simulink model "BlueROV2_Simu"  (R2023b)
settings: Solver=FixedStepAuto  StartTime=0.0  StopTime=60  FixedStep=dt  RelTol=1e-3
values from neighbouring files (symbols this model uses):
  dt = 0.1    [Integrate.m]    (also in init.m; init_NIF.m; init_NIF2.m; init_ODE.m)
  Opt_Ballast_Force = Ballast_Compute(Opt_Ballast_Config)    [init_ballast_checking.m]
  Param = BlueROV2_param()    [Integrate.m]    (also in init.m; init_NIF.m; init_NIF2.m; init_ODE.m)
  tau_b_test = [0; 0; 0; 0; 0; 0]    [init_ballast_checking.m]
  Tether_Force = zeros(6,1)    [Integrate.m]    (also in init.m; init_NIF.m; init_NIF2.m; init_ODE.m)
settings Model: Creator=goks  LastModifiedBy=HP

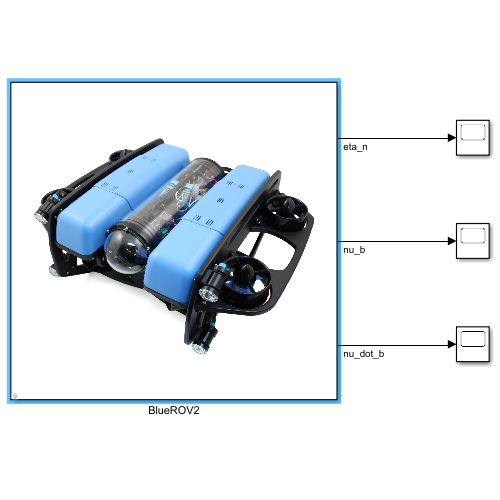
[thumbnail: Simulink's stored preview of the top-level diagram]
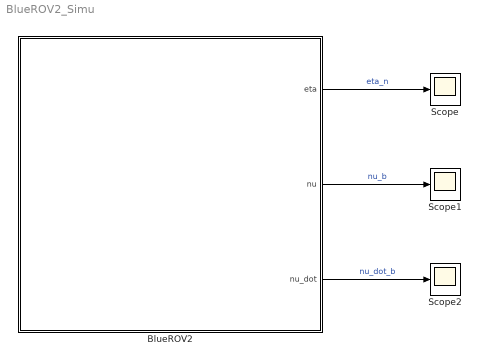
== system BlueROV2_Simu ==
  BlueROV2 : Subsystem
      mask DialogControl DescTextVar Prompt: %<BlueROV2>
      mask Display: image('heavy-bluerov.jpg');
  Scope : Scope
  Scope1 : Scope
  Scope2 : Scope
  wires:
  BlueROV2/1(eta) -> Scope/1  "eta_n"
  BlueROV2/2(nu) -> Scope1/1  "nu_b"
  BlueROV2/3(nu_dot) -> Scope2/1  "nu_dot_b"

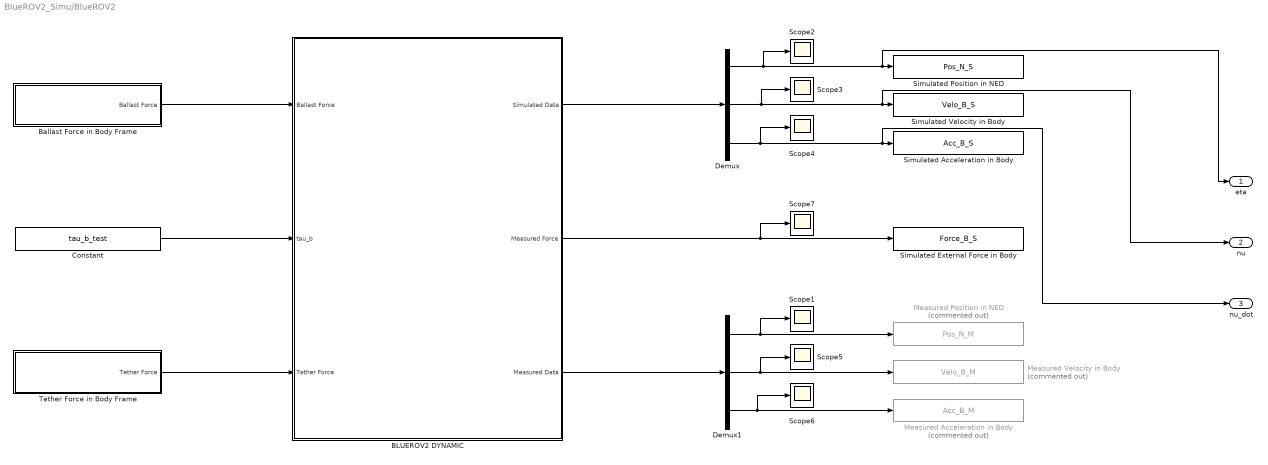
== system BlueROV2_Simu/BlueROV2 ==
  BLUEROV2 DYNAMIC : Subsystem
  Ballast Force in Body Frame : Subsystem
  Constant : Constant  Value=tau_b_test
  Demux : Demux  Outputs=3
  Demux1 : Demux  Outputs=3
  Measured Acceleration in Body : ToWorkspace  Commented=on  VariableName=Acc_B_M  SampleTime=-1
  Measured Position in NED : ToWorkspace  Commented=on  VariableName=Pos_N_M  SampleTime=-1
  Measured Velocity in Body : ToWorkspace  Commented=on  VariableName=Velo_B_M  SampleTime=-1
  Scope{1..7} (7 alike) : Scope
  Simulated Acceleration in Body : ToWorkspace  VariableName=Acc_B_S  SampleTime=-1
  Simulated External Force in Body : ToWorkspace  VariableName=Force_B_S  SampleTime=-1
  Simulated Position in NED : ToWorkspace  VariableName=Pos_N_S  SampleTime=-1
  Simulated Velocity in Body : ToWorkspace  VariableName=Velo_B_S  SampleTime=-1
  Tether Force in Body Frame : Subsystem
  eta : Outport
  nu : Outport  Port=2
  nu_dot : Outport  Port=3
  wires:
  Tether Force in Body Frame/1(Tether Force) -> BLUEROV2 DYNAMIC/3(Tether Force)
  Demux/2 -> Simulated Velocity in Body/1, nu/1, Scope3/1
  BLUEROV2 DYNAMIC/1(Simulated Data) -> Demux/1
  Demux1/1 -> Measured Position in NED/1, Scope1/1
  BLUEROV2 DYNAMIC/3(Measured Data) -> Demux1/1
  Ballast Force in Body Frame/1(Ballast Force) -> BLUEROV2 DYNAMIC/1(Ballast Force)
  Demux/1 -> eta/1, Simulated Position in NED/1, Scope2/1
  Demux1/2 -> Measured Velocity in Body/1, Scope5/1
  Demux1/3 -> Scope6/1, Measured Acceleration in Body/1
  BLUEROV2 DYNAMIC/2(Measured Force) -> Scope7/1, Simulated External Force in Body/1
  Constant/1 -> BLUEROV2 DYNAMIC/2(tau_b)
  Demux/3 -> nu_dot/1, Simulated Acceleration in Body/1, Scope4/1

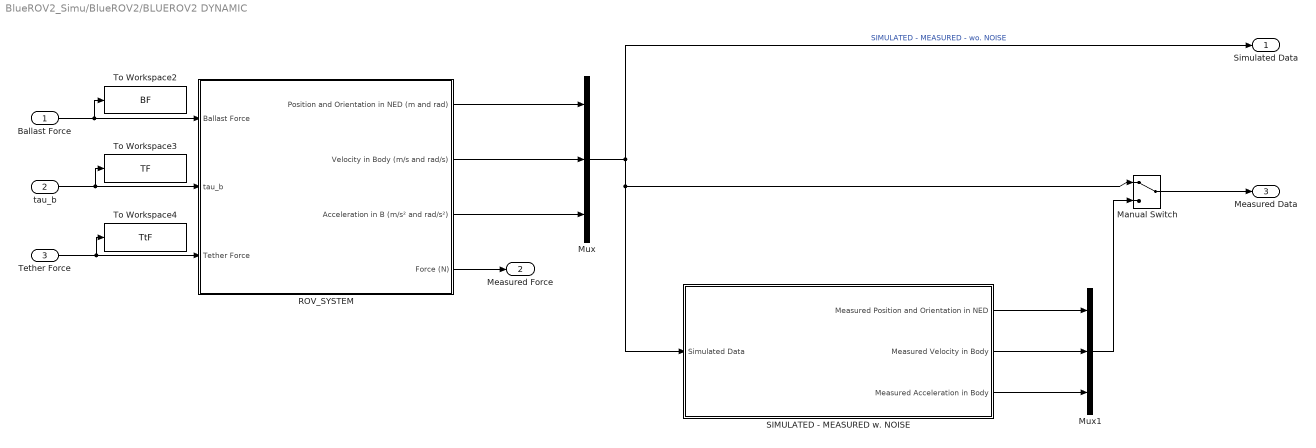
== system BlueROV2_Simu/BlueROV2/BLUEROV2 DYNAMIC ==
  Ballast Force : Inport
  tau_b : Inport  Port=2
  Tether Force : Inport  Port=3
  Manual Switch : ManualSwitch
  Mux : Mux  Inputs=3
  Mux1 : Mux  Inputs=3
  ROV_SYSTEM : Subsystem
  SIMULATED - MEASURED w. NOISE : Subsystem
  To Workspace2 : ToWorkspace  VariableName=BF  SampleTime=-1
  To Workspace3 : ToWorkspace  VariableName=TF  SampleTime=-1
  To Workspace4 : ToWorkspace  VariableName=TtF  SampleTime=-1
  Simulated Data : Outport
  Measured Force : Outport  Port=2
  Measured Data : Outport  Port=3
  wires:
  ROV_SYSTEM/1(Position and Orientation in NED (m and rad)) -> Mux/1
  ROV_SYSTEM/2(Velocity in Body (m/s and rad/s)) -> Mux/2
  ROV_SYSTEM/3(Acceleration in B (m/s² and rad/s²)) -> Mux/3
  ROV_SYSTEM/4(Force (N)) -> Measured Force/1
  SIMULATED - MEASURED w. NOISE/2(Measured Velocity in Body) -> Mux1/2
  SIMULATED - MEASURED w. NOISE/1(Measured Position and Orientation in NED) -> Mux1/1
  SIMULATED - MEASURED w. NOISE/3(Measured Acceleration in Body) -> Mux1/3
  Mux/1 -> SIMULATED - MEASURED w. NOISE/1(Simulated Data), Manual Switch/1, Simulated Data/1  "SIMULATED - MEASURED - wo. NOISE"
  Manual Switch/1 -> Measured Data/1
  Mux1/1 -> Manual Switch/2
  Ballast Force/1 -> ROV_SYSTEM/1(Ballast Force), To Workspace2/1
  tau_b/1 -> ROV_SYSTEM/2(tau_b), To Workspace3/1
  Tether Force/1 -> To Workspace4/1, ROV_SYSTEM/3(Tether Force)

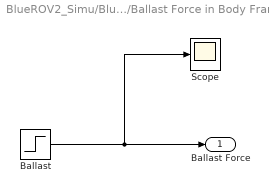
== system BlueROV2_Simu/BlueROV2/Ballast Force in Body Frame ==
  Ballast : Step  Time=0  Before=Opt_Ballast_Force  After=Opt_Ballast_Force  SampleTime=0
  Scope : Scope
  Ballast Force : Outport
  wires:
  Ballast/1 -> Scope/1, Ballast Force/1

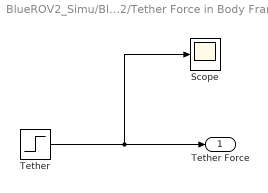
== system BlueROV2_Simu/BlueROV2/Tether Force in Body Frame ==
  Scope : Scope
  Tether : Step  Before=Tether_Force  After=Tether_Force  SampleTime=0
  Tether Force : Outport
  wires:
  Tether/1 -> Scope/1, Tether Force/1

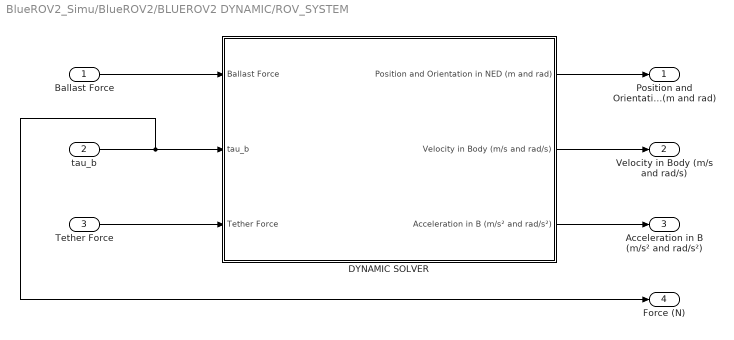
== system BlueROV2_Simu/BlueROV2/BLUEROV2 DYNAMIC/ROV_SYSTEM ==
  Ballast Force : Inport
  tau_b : Inport  Port=2
  Tether Force : Inport  Port=3
  DYNAMIC SOLVER : Subsystem
  Position and Orientation in NED (m and rad) : Outport
  Velocity in Body (m/s and rad/s) : Outport  Port=2
  Acceleration in B (m/s² and rad/s²) : Outport  Port=3
  Force (N) : Outport  Port=4
  wires:
  DYNAMIC SOLVER/2(Velocity in Body (m/s and rad/s)) -> Velocity in Body (m/s and rad/s)/1
  DYNAMIC SOLVER/1(Position and Orientation in NED (m and rad)) -> Position and Orientation in NED (m and rad)/1
  DYNAMIC SOLVER/3(Acceleration in B (m/s² and rad/s²)) -> Acceleration in B (m/s² and rad/s²)/1
  tau_b/1 -> DYNAMIC SOLVER/2(tau_b), Force (N)/1
  Ballast Force/1 -> DYNAMIC SOLVER/1(Ballast Force)
  Tether Force/1 -> DYNAMIC SOLVER/3(Tether Force)

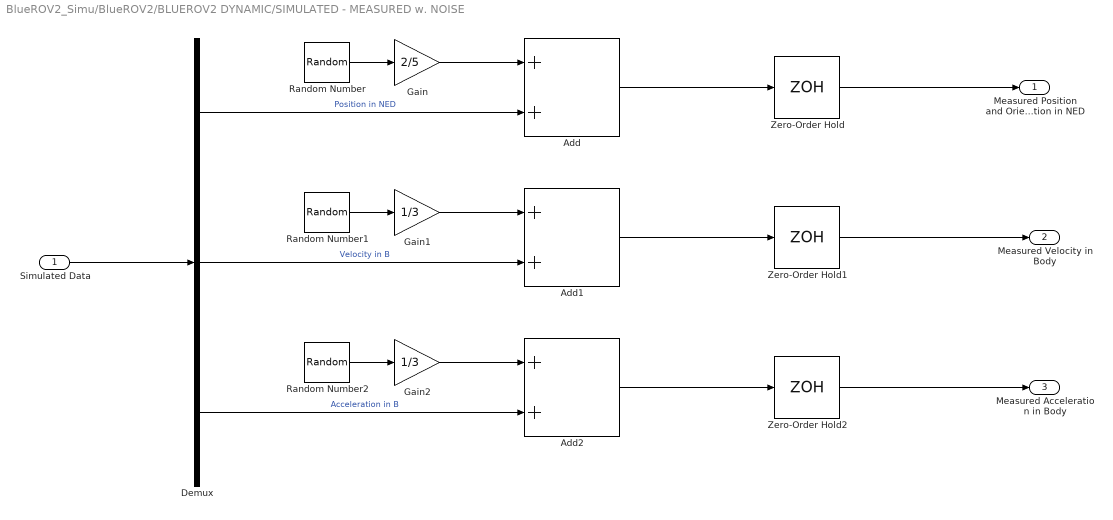
== system BlueROV2_Simu/BlueROV2/BLUEROV2 DYNAMIC/SIMULATED - MEASURED w. NOISE ==
  Simulated Data : Inport
  Add : Sum
  Add1 : Sum
  Add2 : Sum
  Demux : Demux  Outputs=3
  Gain : Gain  Gain=2/5
  Gain1 : Gain  Gain=1/3
  Gain2 : Gain  Gain=1/3
  Random Number : RandomNumber  Variance=0.01  SampleTime=dt
  Random Number1 : RandomNumber  Variance=0.01  SampleTime=dt
  Random Number2 : RandomNumber  Variance=0.01  SampleTime=dt
  Zero-Order Hold : ZeroOrderHold  SampleTime=-1
  Zero-Order Hold1 : ZeroOrderHold  SampleTime=-1
  Zero-Order Hold2 : ZeroOrderHold  SampleTime=-1
  Measured Position and Orientation in NED : Outport
  Measured Velocity in Body : Outport  Port=2
  Measured Acceleration in Body : Outport  Port=3
  wires:
  Simulated Data/1 -> Demux/1
  Demux/1 -> Add/2  "Position in NED"
  Random Number/1 -> Gain/1
  Gain/1 -> Add/1
  Random Number1/1 -> Gain1/1
  Demux/2 -> Add1/2  "Velocity in B"
  Gain1/1 -> Add1/1
  Random Number2/1 -> Gain2/1
  Demux/3 -> Add2/2  "Acceleration in B"
  Gain2/1 -> Add2/1
  Add/1 -> Zero-Order Hold/1
  Add1/1 -> Zero-Order Hold1/1
  Add2/1 -> Zero-Order Hold2/1
  Zero-Order Hold/1 -> Measured Position and Orientation in NED/1
  Zero-Order Hold1/1 -> Measured Velocity in Body/1
  Zero-Order Hold2/1 -> Measured Acceleration in Body/1

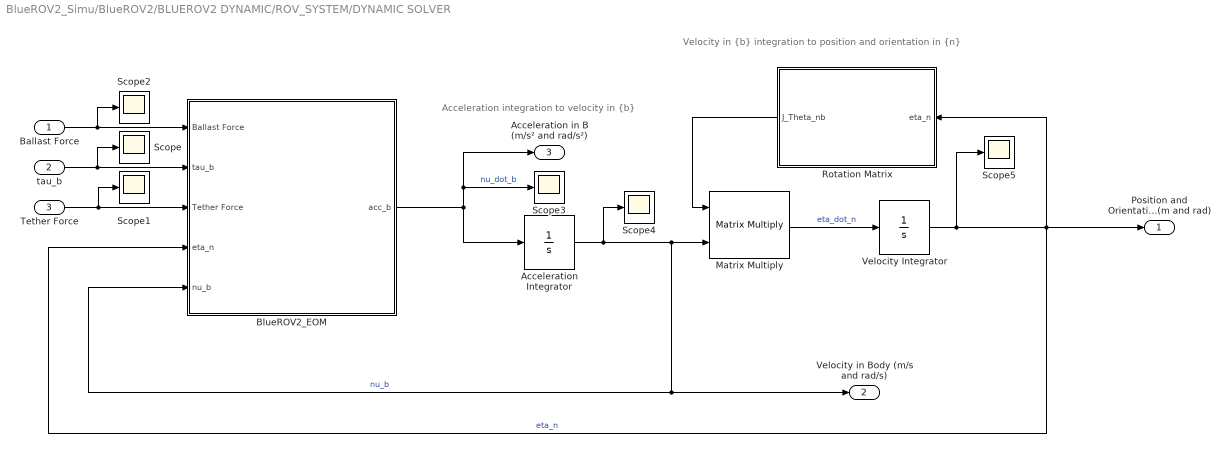
== system BlueROV2_Simu/BlueROV2/BLUEROV2 DYNAMIC/ROV_SYSTEM/DYNAMIC SOLVER ==
  note: Velocity in {b} integration to position and orientation in {n}
  note: Acceleration integration to velocity in {b}
  Ballast Force : Inport
  tau_b : Inport  Port=2
  Tether Force : Inport  Port=3
  Acceleration Integrator : Integrator  InitialCondition=Param.IC.Velo
  BlueROV2_EOM : Subsystem
  Matrix Multiply : Product  Multiplication=Matrix(*)
  Rotation Matrix : MATLAB Function  TreatAsAtomicUnit=on
  Scope{,1..5} (6 alike) : Scope
  Velocity Integrator : Integrator  InitialCondition=Param.IC.Pos
  Position and Orientation in NED (m and rad) : Outport
  Velocity in Body (m/s and rad/s) : Outport  Port=2
  Acceleration in B (m/s² and rad/s²) : Outport  Port=3
  wires:
  tau_b/1 -> BlueROV2_EOM/2(tau_b), Scope/1
  Rotation Matrix/1(J_Theta_nb) -> Matrix Multiply/1
  Matrix Multiply/1 -> Velocity Integrator/1  "eta_dot_n"
  Ballast Force/1 -> Scope2/1, BlueROV2_EOM/1(Ballast Force)
  BlueROV2_EOM/1(acc_b) -> Acceleration Integrator/1, Acceleration in B (m/s² and rad/s²)/1, Scope3/1  "nu_dot_b"
  Tether Force/1 -> BlueROV2_EOM/3(Tether Force), Scope1/1
  Velocity Integrator/1 -> BlueROV2_EOM/4(eta_n), Rotation Matrix/1(eta_n), Position and Orientation in NED (m and rad)/1, Scope5/1  "eta_n"
  Acceleration Integrator/1 -> Scope4/1, BlueROV2_EOM/5(nu_b), Velocity in Body (m/s and rad/s)/1, Matrix Multiply/2  "nu_b"

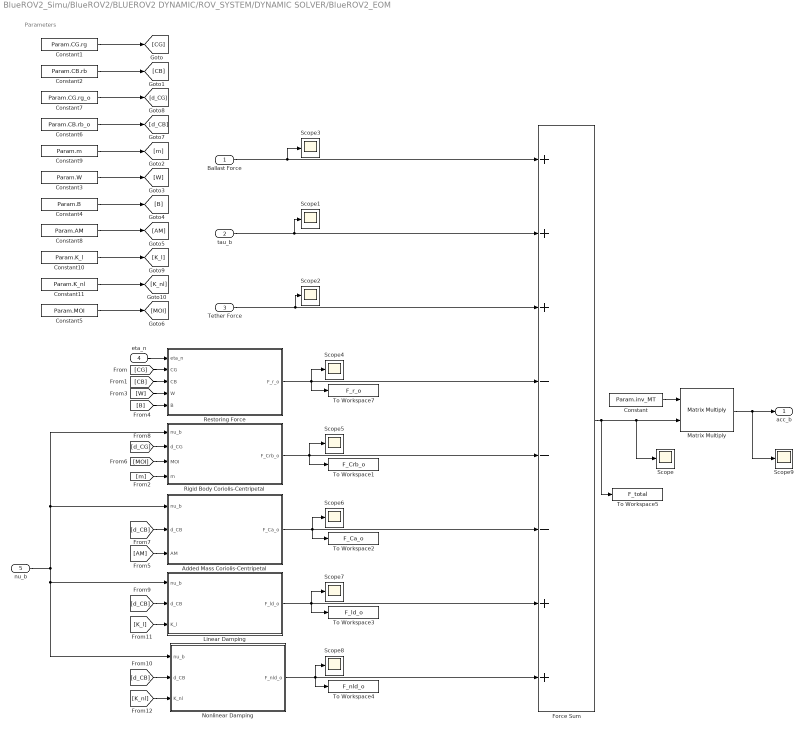
== system BlueROV2_Simu/BlueROV2/BLUEROV2 DYNAMIC/ROV_SYSTEM/DYNAMIC SOLVER/BlueROV2_EOM ==
  note: Parameters
  Ballast Force : Inport
  tau_b : Inport  Port=2
  Tether Force : Inport  Port=3
  eta_n : Inport  Port=4
  nu_b : Inport  Port=5
  Added Mass Coriolis-Centripetal : MATLAB Function  TreatAsAtomicUnit=on
  Constant : Constant  Value=Param.inv_MT
  Constant1 : Constant  Value=Param.CG.rg
  Constant10 : Constant  Value=Param.K_l
  Constant11 : Constant  Value=Param.K_nl
  Constant2 : Constant  Value=Param.CB.rb
  Constant3 : Constant  Value=Param.W
  Constant4 : Constant  Value=Param.B
  Constant5 : Constant  Value=Param.MOI
  Constant6 : Constant  Value=Param.CB.rb_o
  Constant7 : Constant  Value=Param.CG.rg_o
  Constant8 : Constant  Value=Param.AM
  Constant9 : Constant  Value=Param.m
  Force Sum : Sum  Inputs=+++---++
  Linear Damping : MATLAB Function  TreatAsAtomicUnit=on
  Matrix Multiply : Product  Multiplication=Matrix(*)
  Nonlinear Damping : MATLAB Function  TreatAsAtomicUnit=on
  Restoring Force : MATLAB Function  TreatAsAtomicUnit=on
  Rigid Body Coriolis-Centripetal : MATLAB Function  TreatAsAtomicUnit=on
  Scope{,1..9} (10 alike) : Scope
  To Workspace1 : ToWorkspace  VariableName=F_Crb_o  SampleTime=-1
  To Workspace2 : ToWorkspace  VariableName=F_Ca_o  SampleTime=-1
  To Workspace3 : ToWorkspace  VariableName=F_ld_o  SampleTime=-1
  To Workspace4 : ToWorkspace  VariableName=F_nld_o  SampleTime=-1
  To Workspace5 : ToWorkspace  VariableName=F_total  SampleTime=-1
  To Workspace7 : ToWorkspace  VariableName=F_r_o  SampleTime=-1
  acc_b : Outport
  wires:
  eta_n/1 -> Restoring Force/1(eta_n)
  nu_b/1 -> Nonlinear Damping/1(nu_b), Linear Damping/1(nu_b), Rigid Body Coriolis-Centripetal/1(nu_b), Added Mass Coriolis-Centripetal/1(nu_b)
  Force Sum/1 -> To Workspace5/1, Scope/1, Matrix Multiply/2
  Constant/1 -> Matrix Multiply/1
  Matrix Multiply/1 -> Scope9/1, acc_b/1
  Ballast Force/1 -> Scope3/1, Force Sum/1
  tau_b/1 -> Scope1/1, Force Sum/2
  Tether Force/1 -> Scope2/1, Force Sum/3
  Restoring Force/1(F_r_o) -> To Workspace7/1, Force Sum/4, Scope4/1
  Rigid Body Coriolis-Centripetal/1(F_Crb_o) -> Scope5/1, To Workspace1/1, Force Sum/5
  Added Mass Coriolis-Centripetal/1(F_Ca_o) -> To Workspace2/1, Scope6/1, Force Sum/6
  Linear Damping/1(F_ld_o) -> To Workspace3/1, Scope7/1, Force Sum/7
  Nonlinear Damping/1(F_nld_o) -> Scope8/1, To Workspace4/1, Force Sum/8
  Constant1/1 -> [CG]
  Constant2/1 -> [CB]
  Constant6/1 -> [d_CB]
  Constant7/1 -> [d_CG]
  Constant9/1 -> [m]
  Constant3/1 -> [W]
  Constant4/1 -> [B]
  Constant8/1 -> [AM]
  Constant5/1 -> [MOI]
  [CG] -> Restoring Force/2(CG)
  [CB] -> Restoring Force/3(CB)
  [W] -> Restoring Force/4(W)
  [B] -> Restoring Force/5(B)
  [d_CG] -> Rigid Body Coriolis-Centripetal/2(d_CG)
  [m] -> Rigid Body Coriolis-Centripetal/4(m)
  [MOI] -> Rigid Body Coriolis-Centripetal/3(MOI)
  [d_CB] -> Added Mass Coriolis-Centripetal/2(d_CB)
  [AM] -> Added Mass Coriolis-Centripetal/3(AM)
  [d_CB] -> Linear Damping/2(d_CB)
  [d_CB] -> Nonlinear Damping/2(d_CB)
  [K_l] -> Linear Damping/3(K_l)
  [K_nl] -> Nonlinear Damping/3(K_nl)
  Constant10/1 -> [K_l]
  Constant11/1 -> [K_nl]

== matlab function BlueROV2_Simu/BlueROV2/BLUEROV2 DYNAMIC/ROV_SYSTEM/DYNAMIC SOLVER/BlueROV2_EOM/Restoring Force ==
  data: eta_n input; F_r_o output; CG input; CB input; W input; B input
function F_r_o   = Restoring_Force(eta_n, CG, CB, W, B)
%% Restoring Forces
% Described in Body Frame, at Center of Gravity. ALREADY FOR THE LEFT HAND SIDE
% Orientation
phi = eta_n(4);
theta = eta_n(5);

% Gravity
xg = CG(1);
yg = CG(2);
zg = CG(3);

% Buoyancy
xb = CB(1);
yb = CB(2);
zb = CB(3);

% % Force
% Fg_n = [0; 0; W];
% Fb_n = -[0; 0; B];
% 
% F_r_o = -[Rot_bn(eta_n) * Fg_n + Rot_bn(eta_n) * Fb_n;
%          cross(CG, Rot_bn(eta_n) * Fg_n) + cross(CB, Rot_bn(eta_n) * Fb_n)];

% Force
F_r_o = [(W - B)*sin(theta);
         -(W - B)*cos(theta)*sin(phi);
         -(W - B)*cos(theta)*cos(phi);
         -(yg*W - yb*B)*cos(theta)*cos(phi) + (zg*W - zb*B)*cos(theta)*sin(phi);
         (zg*W - zb*B)*sin(theta) + (xg*W - xb*B)*cos(theta)*cos(phi);
         -(xg*W - xb*B)*cos(theta)*sin(phi) - (yg*W - yb*B)*sin(theta)];

% For debugging
% F_r_o = zeros(6,1);
end

== matlab function BlueROV2_Simu/BlueROV2/BLUEROV2 DYNAMIC/ROV_SYSTEM/DYNAMIC SOLVER/Rotation Matrix ==
  data: eta_n input; J_Theta_nb output
function J_Theta_nb = Transform_nb(eta_n)
%%%%%%%%%%%%%%%%%%%%%%%%%%%%%%%%%%%%%%%%%%%%%%%%%%%%%%%%%%%%%%%%%%%%%%%%%%%
% Command                                                                 %
%                                                                         %
% Compute the Jacobian from {b} to {n}                                    %
%                                                                         %
% For 6-DOF Equations:                                                    %
% [ndot = Jacobian(n_theta) * v]                                          %
% -ndot = velocity expressed in NED frame                                 %
% -n_theta = rotational part of position vector                           %
% - v = velocity expressed in Body frame                                  %
%                                                                         %
% Argument:                                                               %
% eta     : Input positional vector                                       %
%                                                                         %
% Created:      27.09.2023	Andreas Sitorus                               %
%                                                                         %
%%%%%%%%%%%%%%%%%%%%%%%%%%%%%%%%%%%%%%%%%%%%%%%%%%%%%%%%%%%%%%%%%%%%%%%%%%%
%% Get the orientation
phi = eta_n(4,1);       % Rolling angle
theta = eta_n(5,1);     % Pitching angle
psi = eta_n(6,1);       % Yaw angle

%% Linear Velocity Transformation Matrix
% Element
r11 = cos(psi) * cos(theta);
r12 = -sin(psi) * cos(phi) + cos(psi) * sin(theta) * sin(phi);
r13 = sin(psi) * sin(phi) + cos(psi) * cos(phi) * sin(theta);
r21 = sin(psi) * cos(theta);
r22 = cos(psi) * cos(phi) + sin(phi) * sin(theta) * sin(psi);
r23 = -cos(psi) * sin(phi) + sin(theta) * sin(psi) * cos(phi);
r31 = -sin(theta);
r32 = cos(theta) * sin(phi);
r33 = cos(theta) * cos(phi);

% Rotation Matrix (from {b} to {n})
R_Theta_nb = [r11 r12 r13;
              r21 r22 r23;
              r31 r32 r33];

%% Angular Velocity Transformation Matrix
% Element
t11 = 1;
t12 = sin(phi) * tan(theta);
t13 = cos(phi) * tan(theta);
t21 = 0;
t22 = cos(phi);
t23 = -sin(phi);
t31 = 0;
t32 = sin(phi) / cos(theta);
t33 = cos(phi) / cos(theta);

% Angular Velocity Rotation Matrix (from {b} to {n})
T_Theta_nb = [t11 t12 t13;
              t21 t22 t23;
              t31 t32 t33];

%% Jacobian
J_Theta_nb = [R_Theta_nb  zeros(3);
              zeros(3) T_Theta_nb];

end

== matlab function BlueROV2_Simu/BlueROV2/BLUEROV2 DYNAMIC/ROV_SYSTEM/DYNAMIC SOLVER/BlueROV2_EOM/Rigid Body Coriolis-Centripetal ==
  data: nu_b input; F_Crb_o output; d_CG input; MOI input; m input
function F_Crb_o    = Coriolis_Centripetal_RB_Force(nu_b, d_CG, MOI, m)
%% Coriolis-Centripetal Forces
% % Velocity
% u = nu_b(1);
% v = nu_b(2);
% w = nu_b(3);
% p = nu_b(4);
% q = nu_b(5);
% r = nu_b(6);

% Distance from CG to CO
% Defined as d_CG

% Transformed Velocity
V_t_g = H_(-d_CG) * nu_b;  % 6DOF Velocity, expressed in CG

% Get CoG-body velocity
u_cg = V_t_g(1,1);
v_cg = V_t_g(2,1);
w_cg = V_t_g(3,1);
p_cg = V_t_g(4,1);
q_cg = V_t_g(5,1);
r_cg = V_t_g(6,1);

% MOI
Ixx = MOI(1);
Iyy = MOI(2);
Izz = MOI(3);

% CC-Rigid Body
% Described in Body frame, at Center of Gravity

Crb11 = zeros(3); 
Crb12 = [0 m*w_cg -m*v_cg;
         -m*w_cg 0 m*u_cg;
         m*v_cg -m*u_cg 0];
Crb21 = Crb12;
Crb22 = [0 -Izz*r_cg -Iyy*q_cg;
         Izz*r_cg 0 Ixx*p_cg;
         Iyy*q_cg -Ixx*p_cg 0];

Crb = [Crb11 Crb12;
       Crb21 Crb22]; % Rigid Body Coriolis Force Matrix, at Center of Gravity

% Force
F_Crb_o = (H_(d_CG))' * Crb * V_t_g;

% For debugging
% F_Crb_o = Crb * nu_b;
% F_Crb_o = zeros(6,1);
end

== matlab function BlueROV2_Simu/BlueROV2/BLUEROV2 DYNAMIC/ROV_SYSTEM/DYNAMIC SOLVER/BlueROV2_EOM/Added Mass Coriolis-Centripetal ==
  data: nu_b input; F_Ca_o output; d_CB input; AM input
function F_Ca_o    = Coriolis_Centripetal_AM_Force(nu_b, d_CB, AM)
%% Coriolis-Centripetal Forces
% % Velocity
% u = nu_b(1);
% v = nu_b(2);
% w = nu_b(3);
% p = nu_b(4);
% q = nu_b(5);
% r = nu_b(6);

% Distance from CB to CO
% Defined as d_CB

% Transformed Velocity
V_t_b = H_(-d_CB) * nu_b;  % 6DOF Velocity, expressed in CB

% Get CoB-body velocity
u_cb = V_t_b(1,1);
v_cb = V_t_b(2,1);
w_cb = V_t_b(3,1);
p_cb = V_t_b(4,1);
q_cb = V_t_b(5,1);
r_cb = V_t_b(6,1);

% Added Mass Coefficient
Xud = AM(1);
Yvd = AM(2);
Zwd = AM(3);
Kpd = AM(4);
Mqd = AM(5);
Nrd = AM(6);

% CC-Added Mass
% Described in Body frame, at Center of Buoyancy
Ca11 = zeros(3);
Ca12 = [0 -Zwd*w_cb Yvd*v_cb;
        Zwd*w_cb 0 -Xud*u_cb;
        -Yvd*v_cb Xud*u_cb 0];
Ca21 = Ca12;
Ca22 = [0 -Nrd*r_cb Mqd*q_cb;
        Nrd*r_cb 0 -Kpd*p_cb;
        -Mqd*q_cb Kpd*p_cb 0];

Ca = [Ca11 Ca12;
      Ca21 Ca22]; % Added mass Coriolis Force Matrix, at Center of Buoyancy

% Force
F_Ca_o = (H_(d_CB))' * Ca * V_t_b;

% For debugging
% F_Ca_o = Ca * nu_b;
% F_Ca_o = zeros(6,1);
end

== matlab function BlueROV2_Simu/BlueROV2/BLUEROV2 DYNAMIC/ROV_SYSTEM/DYNAMIC SOLVER/BlueROV2_EOM/Linear Damping ==
  data: F_ld_o output; nu_b input; d_CB input; K_l input
function F_ld_o  = Linear_Damping(nu_b, d_CB, K_l)
% %% Linear Damping Forces
% % Distance from CB to CO
% % Defined as d_CB

% Transformed Velocity
V_t_b = H_(-d_CB) * nu_b;  % 6DOF Velocity, expressed in CB

% Force
F_ld_o = -(H_(d_CB))' * diag(K_l) * V_t_b; 

% For debugging
% F_ld_o = -diag(L_Damping_Matrix) * nu_b; 
% F_ld_o = zeros(6,1); 
end

== matlab function BlueROV2_Simu/BlueROV2/BLUEROV2 DYNAMIC/ROV_SYSTEM/DYNAMIC SOLVER/BlueROV2_EOM/Nonlinear Damping ==
  data: F_nld_o output; nu_b input; d_CB input; K_nl input
function F_nld_o = Nonlinear_Damping_forces(nu_b, d_CB, K_nl)
%% Nonlinear Damping Forces
% Velocity
u = nu_b(1);
v = nu_b(2);
w = nu_b(3);
p = nu_b(4);
q = nu_b(5);
r = nu_b(6);

% Distance from CB to CO
% Defined as d_CB

% Transformed Velocity
V_t_b = H_(-d_CB) * nu_b;  % 6DOF Velocity, expressed in CB

% Nonlinear Damping Matrix
NL_Damping_Coeff = diag(K_nl) * abs(V_t_b);

% Force
F_nld_o = -(H_(d_CB))' * diag(NL_Damping_Coeff) * V_t_b;

% For debugging
% F_nld_o = -diag(NL_Damping_Coeff) * nu_b;
% F_nld_o = zeros(6,1);
end
